simulink model "model_full"  (R2021b)
settings: Solver=VariableStepAuto  StartTime=0.0  StopTime=T  FixedStep=0.001  RelTol=1e-3
undefined symbols (not defined in the file): D, dz_width, i0, J, ke, L, R, U, v0
settings Model: Creator=mateusz  LastModifiedBy=mateusz
settings SolverCC: ZeroCrossAlgorithm=Adaptive
settings DebuggingCC: IgnoredZcDiagnostic=none

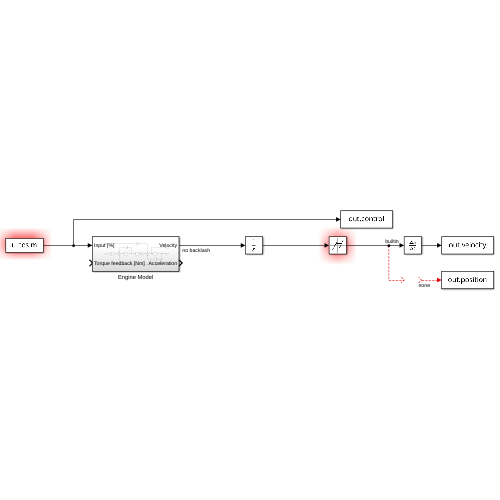
[thumbnail: Simulink's stored preview of the top-level diagram]
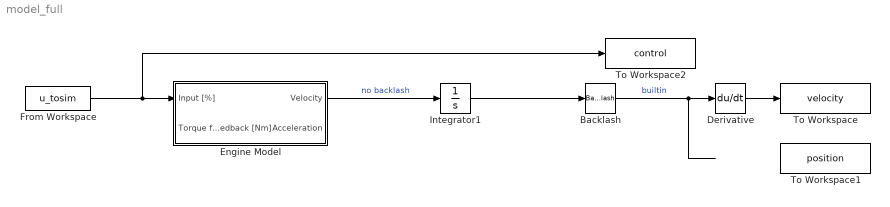
== system model_full ==
  Backlash : Backlash  BacklashWidth=b_width
  Derivative : Derivative
  Engine Model : Subsystem
  From Workspace : FromWorkspace  VariableName=u_tosim
  Integrator1 : Integrator
  To Workspace : ToWorkspace  VariableName=velocity  SaveFormat=Structure With Time  SampleTime=-1
  To Workspace1 : ToWorkspace  VariableName=position  SaveFormat=Structure With Time  SampleTime=-1
  To Workspace2 : ToWorkspace  VariableName=control  SaveFormat=Structure With Time  SampleTime=-1
  wires:
  From Workspace/1 -> To Workspace2/1, Engine Model/1(Input [%])
  Backlash/1 -> Derivative/1  "builtin"
  ? -> To Workspace1/1  "none"
  Engine Model/1(Velocity) -> Integrator1/1  "no backlash"
  Integrator1/1 -> Backlash/1
  Derivative/1 -> To Workspace/1

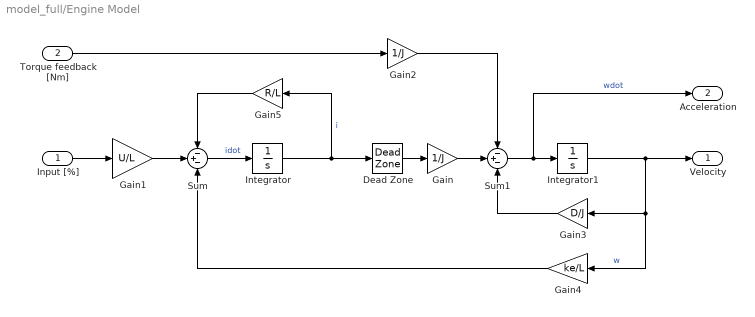
== system model_full/Engine Model ==
  Input [%] : Inport
  Torque feedback [Nm] : Inport  Port=2
  Dead Zone : DeadZone  LowerValue=-dz_width  UpperValue=dz_width  SaturateOnIntegerOverflow=on
  Gain : Gain  Gain=1/J
  Gain1 : Gain  Gain=U/L
  Gain2 : Gain  Gain=1/J
  Gain3 : Gain  Gain=D/J
  Gain4 : Gain  Gain=ke/L
  Gain5 : Gain  Gain=R/L
  Integrator : Integrator  InitialCondition=i0
  Integrator1 : Integrator  InitialCondition=v0
  Sum : Sum  Inputs=-+-
  Sum1 : Sum  Inputs=-+-
  Velocity : Outport
  Acceleration : Outport  Port=2
  wires:
  Gain3/1 -> Sum1/3
  Input [%]/1 -> Gain1/1
  Gain4/1 -> Sum/3
  Dead Zone/1 -> Gain/1
  Gain/1 -> Sum1/2
  Gain5/1 -> Sum/1
  Sum/1 -> Integrator/1  "idot"
  Gain1/1 -> Sum/2
  Sum1/1 -> Acceleration/1, Integrator1/1  "wdot"
  Integrator/1 -> Gain5/1, Dead Zone/1  "i"
  Integrator1/1 -> Velocity/1, Gain4/1, Gain3/1  "w"
  Torque feedback [Nm]/1 -> Gain2/1
  Gain2/1 -> Sum1/1
